simulink model "rc_coder"  (R2019b)
settings: Solver=FixedStepDiscrete  StartTime=0.0  StopTime=Inf  FixedStep=0.025  RelTol=1e-3  EnableMultiTasking=on
PreLoadFcn:
  | mdlname = bdroot;
  | oldFolder = cd(fileparts(which(mdlname)));
  | % cd ..\
  | 
  | load('./bus_type/bus_type.mat');
model workspace (MAT data in the model file):
  ADCDRES : Simulink.Parameter (value not decoded)
  ADCSRES : Simulink.Parameter (value not decoded)
  CLK : Simulink.Parameter (value not decoded)
  EncoderScaler : Simulink.Parameter (value not decoded)
  GearBoxScaler : Simulink.Parameter (value not decoded)
  Kd_T : Simulink.Parameter (value not decoded)
  Kd_theta : Simulink.Parameter (value not decoded)
  Ki_T : Simulink.Parameter (value not decoded)
  Ki_theta : Simulink.Parameter (value not decoded)
  Kp_T : Simulink.Parameter (value not decoded)
  Kp_theta : Simulink.Parameter (value not decoded)
  LowerTempLimitHigh : Simulink.Parameter (value not decoded)
  LowerTempLimitLow : Simulink.Parameter (value not decoded)
  MinMeasurableSpd : Simulink.Parameter (value not decoded)
  ModePWM : Simulink.Parameter (value not decoded)
  ModePosition : Simulink.Parameter (value not decoded)
  ModePrecool : Simulink.Parameter (value not decoded)
  ModeTemp : Simulink.Parameter (value not decoded)
  PWMFreq : Simulink.Parameter (value not decoded)
  QuadratureEncScaler : Simulink.Parameter (value not decoded)
  S1DelaySeconds : Simulink.Parameter (value not decoded)
  S2DelaySeconds : Simulink.Parameter (value not decoded)
  S3DelaySeconds : Simulink.Parameter (value not decoded)
  S4DelaySeconds : Simulink.Parameter (value not decoded)
  SamplingR : Simulink.Parameter (value not decoded)
  StepSize : Simulink.Parameter (value not decoded)
  TErrBand : Simulink.Parameter (value not decoded)
  ThetaErrBand : Simulink.Parameter (value not decoded)
  VADCREF : Simulink.Parameter (value not decoded)
symbols that are objects in the model workspace (value not decoded): ADCDRES, CLK, EncoderScaler, GearBoxScaler, Kd_T, Kd_theta, Ki_T, Ki_theta, Kp_T, Kp_theta, LowerTempLimitHigh, LowerTempLimitLow, MinMeasurableSpd, ModePosition, ModePrecool, ModePWM, ModeTemp, PWMFreq, QuadratureEncScaler, S1DelaySeconds, S2DelaySeconds, S3DelaySeconds, S4DelaySeconds, StepSize, TErrBand, ThetaErrBand
undefined symbols (not defined in the file or in its folder): DiscIntNeverNeededParam, Down, GPTRIP1SEL, GPTRIP2SEL, TZ1, TZ2, Up
libraries: simulink x21, c2802xlib x12, c2837xDlib x10, c280xlib x9, dspstat3 x8, dspfdesign x7, commutil2 x3, c2000lib x2
(part 3 of 4)

== system rc_coder/Sensing/Temperature Measurement/Subsystem ==
  In1 : Inport
  In2 : Inport  Port=2
  In3 : Inport  Port=3
  Divide : Product  Inputs=*/
  Product : Product
  R vs. T : Lookup_n-D  NumberOfTableDimensions=1  BreakpointsForDimension1=|  Table=fliplr([-40:125])  InternalRulePriority=Speed  RndMeth=Simplest  InputSameDT=on
      | flipud([336103
      | 314558
      | 294529
      | 275901
      | 258567
      | 242430
      | 227401
      | 213397
      | 200341
      | 188166
      | 176805
      | 166200
      | 156296
      | 147043
      | 138395
      | 130308
      | 122742
      | 115662
      | 109033
      | 102825
      | 97006.9000000000
      | 91553.3000000000
      | 86439.2000000000
      | 81641.4000000000
      | 77138.6000000000
      | 72911.1000000000
      | 68940.4000000000
      | 65209.7000000000
      | 61702.9000000000
      | 58405.5000000000
      | 55303.9000000000
      | 52385.2000000000
      | 49637.8000000000
      | 47050.6000000000
      | 44613.4000000000
      | 42316.7000000000
      | 40151.6000000000
      | 38110
      | 36184
      | 34366.6000000000
      | 32650.9000000000
      | 31030.8000000000
      | 29500.5000000000
      | 28054.4000000000
      | 26687.5000000000
      | 25395
      | 24172.5000000000
      | 23015.9000000000
      | 21921.2000000000
      | 20884.7000000000
      | 19903.2000000000
      | 18973.3000000000
      | 18092.2000000000
      | 17256.9000000000
      | 16464.9000000000
      | 15713.7000000000
      | 15000.9000000000
      | 14324.5000000000
      | 13682.3000000000
      | 13072.6000000000
      | 12493.3000000000
      | 11943
      | 11419.9000000000
      | 10922.7000000000
      | 10449.8000000000
      | 10000
      | 9572
      | 9164.70000000000
      | 8777
      | 8407.70000000000
      | 8056.10000000000
      | 7721
      | 7401.70000000000
      | 7097.30000000000
      | 6807.10000000000
      | 6530.30000000000
      | 6266.20000000000
      | 6014.30000000000
      | 5773.80000000000
      | 5544.20000000000
      | 5325
      | 5115.60000000000
      | 4915.60000000000
      | 4724.40000000000
      | 4541.70000000000
      | 4367
      | 4200
      | 4040.20000000000
      | 3887.40000000000
      | 3741.10000000000
      | 3601.10000000000
      | 3467
      | 3338.70000000000
      | 3215.80000000000
      | 3098
      | 2985.20000000000
      | 2877
      | 2773.30000000000
      | 2673.90000000000
      | 2578.60000000000
      | 2487.10000000000
      | 2399.40000000000
      | 2315.20000000000
      | 2234.40000000000
      | 2156.80000000000
      | 2082.30000000000
      | 2010.80000000000
      | 1942.10000000000
      | 1876
      | 1812.60000000000
      | 1751.60000000000
      | 1693
      | 1636.60000000000
      | 1582.40000000000
      | 1530.20000000000
      | 1480.10000000000
      | 1431.80000000000
      | 1385.30000000000
      | 1340.60000000000
      | 1297.50000000000
      | 1256.10000000000
      | 1216.10000000000
      | 1177.70000000000
      | 1140.60000000000
      | 1104.90000000000
      | 1070.50000000000
      | 1037.30000000000
      | 1005.30000000000
      | 974.400000000000
      | 944.700000000000
      | 916
      | 888.300000000000
      | 861.500000000000
      | 835.800000000000
      | 810.900000000000
      | 786.800000000000
      | 763.600000000000
      | 741.200000000000
      | 719.600000000000
      | 698.600000000000
      | 678.400000000000
      | 658.900000000000
      | 640
      | 621.800000000000
      | 604.200000000000
      | 587.100000000000
      | 570.600000000000
      | 554.600000000000
      | 539.200000000000
      | 524.300000000000
      | 509.800000000000
      | 495.900000000000
      | 482.300000000000
      | 469.200000000000
      | 456.500000000000
      | 444.200000000000
      | 432.300000000000
      | 420.800000000000
      | 409.700000000000
      | 398.800000000000
      | 388.400000000000
      | 378.200000000000
      | 368.300000000000
      | 358.800000000000
      | 349.500000000000
      | 340.600000000000])
  Subtract : Sum  Inputs=+-
  Out1 : Outport
  wires:
  Product/1 -> Divide/1
  Subtract/1 -> Divide/2
  In3/1 -> Product/2, Subtract/2
  In1/1 -> Subtract/1
  R vs. T/1 -> Out1/1
  In2/1 -> Product/1
  Divide/1 -> R vs. T/1

== system rc_coder/Sensing/Temperature Measurement/Subsystem1 ==
  In1 : Inport
  In2 : Inport  Port=2
  In3 : Inport  Port=3
  Divide : Product  Inputs=*/
  Product : Product
  R vs. T : Lookup_n-D  NumberOfTableDimensions=1  BreakpointsForDimension1=|  Table=fliplr([-40:125])  InternalRulePriority=Speed  RndMeth=Simplest  InputSameDT=on
      | flipud([336103
      | 314558
      | 294529
      | 275901
      | 258567
      | 242430
      | 227401
      | 213397
      | 200341
      | 188166
      | 176805
      | 166200
      | 156296
      | 147043
      | 138395
      | 130308
      | 122742
      | 115662
      | 109033
      | 102825
      | 97006.9000000000
      | 91553.3000000000
      | 86439.2000000000
      | 81641.4000000000
      | 77138.6000000000
      | 72911.1000000000
      | 68940.4000000000
      | 65209.7000000000
      | 61702.9000000000
      | 58405.5000000000
      | 55303.9000000000
      | 52385.2000000000
      | 49637.8000000000
      | 47050.6000000000
      | 44613.4000000000
      | 42316.7000000000
      | 40151.6000000000
      | 38110
      | 36184
      | 34366.6000000000
      | 32650.9000000000
      | 31030.8000000000
      | 29500.5000000000
      | 28054.4000000000
      | 26687.5000000000
      | 25395
      | 24172.5000000000
      | 23015.9000000000
      | 21921.2000000000
      | 20884.7000000000
      | 19903.2000000000
      | 18973.3000000000
      | 18092.2000000000
      | 17256.9000000000
      | 16464.9000000000
      | 15713.7000000000
      | 15000.9000000000
      | 14324.5000000000
      | 13682.3000000000
      | 13072.6000000000
      | 12493.3000000000
      | 11943
      | 11419.9000000000
      | 10922.7000000000
      | 10449.8000000000
      | 10000
      | 9572
      | 9164.70000000000
      | 8777
      | 8407.70000000000
      | 8056.10000000000
      | 7721
      | 7401.70000000000
      | 7097.30000000000
      | 6807.10000000000
      | 6530.30000000000
      | 6266.20000000000
      | 6014.30000000000
      | 5773.80000000000
      | 5544.20000000000
      | 5325
      | 5115.60000000000
      | 4915.60000000000
      | 4724.40000000000
      | 4541.70000000000
      | 4367
      | 4200
      | 4040.20000000000
      | 3887.40000000000
      | 3741.10000000000
      | 3601.10000000000
      | 3467
      | 3338.70000000000
      | 3215.80000000000
      | 3098
      | 2985.20000000000
      | 2877
      | 2773.30000000000
      | 2673.90000000000
      | 2578.60000000000
      | 2487.10000000000
      | 2399.40000000000
      | 2315.20000000000
      | 2234.40000000000
      | 2156.80000000000
      | 2082.30000000000
      | 2010.80000000000
      | 1942.10000000000
      | 1876
      | 1812.60000000000
      | 1751.60000000000
      | 1693
      | 1636.60000000000
      | 1582.40000000000
      | 1530.20000000000
      | 1480.10000000000
      | 1431.80000000000
      | 1385.30000000000
      | 1340.60000000000
      | 1297.50000000000
      | 1256.10000000000
      | 1216.10000000000
      | 1177.70000000000
      | 1140.60000000000
      | 1104.90000000000
      | 1070.50000000000
      | 1037.30000000000
      | 1005.30000000000
      | 974.400000000000
      | 944.700000000000
      | 916
      | 888.300000000000
      | 861.500000000000
      | 835.800000000000
      | 810.900000000000
      | 786.800000000000
      | 763.600000000000
      | 741.200000000000
      | 719.600000000000
      | 698.600000000000
      | 678.400000000000
      | 658.900000000000
      | 640
      | 621.800000000000
      | 604.200000000000
      | 587.100000000000
      | 570.600000000000
      | 554.600000000000
      | 539.200000000000
      | 524.300000000000
      | 509.800000000000
      | 495.900000000000
      | 482.300000000000
      | 469.200000000000
      | 456.500000000000
      | 444.200000000000
      | 432.300000000000
      | 420.800000000000
      | 409.700000000000
      | 398.800000000000
      | 388.400000000000
      | 378.200000000000
      | 368.300000000000
      | 358.800000000000
      | 349.500000000000
      | 340.600000000000])
  Subtract : Sum  Inputs=+-
  Out1 : Outport
  wires:
  Divide/1 -> R vs. T/1
  In2/1 -> Product/1
  R vs. T/1 -> Out1/1
  In1/1 -> Subtract/1
  In3/1 -> Subtract/2, Product/2
  Subtract/1 -> Divide/2
  Product/1 -> Divide/1

== system rc_coder/Sensing/Temperature Measurement/Subsystem2 ==
  In1 : Inport
  In2 : Inport  Port=2
  In3 : Inport  Port=3
  Divide : Product  Inputs=*/
  Product : Product
  R vs. T : Lookup_n-D  NumberOfTableDimensions=1  BreakpointsForDimension1=|  Table=fliplr([-40:125])  InternalRulePriority=Speed  RndMeth=Simplest  InputSameDT=on
      | flipud([336103
      | 314558
      | 294529
      | 275901
      | 258567
      | 242430
      | 227401
      | 213397
      | 200341
      | 188166
      | 176805
      | 166200
      | 156296
      | 147043
      | 138395
      | 130308
      | 122742
      | 115662
      | 109033
      | 102825
      | 97006.9000000000
      | 91553.3000000000
      | 86439.2000000000
      | 81641.4000000000
      | 77138.6000000000
      | 72911.1000000000
      | 68940.4000000000
      | 65209.7000000000
      | 61702.9000000000
      | 58405.5000000000
      | 55303.9000000000
      | 52385.2000000000
      | 49637.8000000000
      | 47050.6000000000
      | 44613.4000000000
      | 42316.7000000000
      | 40151.6000000000
      | 38110
      | 36184
      | 34366.6000000000
      | 32650.9000000000
      | 31030.8000000000
      | 29500.5000000000
      | 28054.4000000000
      | 26687.5000000000
      | 25395
      | 24172.5000000000
      | 23015.9000000000
      | 21921.2000000000
      | 20884.7000000000
      | 19903.2000000000
      | 18973.3000000000
      | 18092.2000000000
      | 17256.9000000000
      | 16464.9000000000
      | 15713.7000000000
      | 15000.9000000000
      | 14324.5000000000
      | 13682.3000000000
      | 13072.6000000000
      | 12493.3000000000
      | 11943
      | 11419.9000000000
      | 10922.7000000000
      | 10449.8000000000
      | 10000
      | 9572
      | 9164.70000000000
      | 8777
      | 8407.70000000000
      | 8056.10000000000
      | 7721
      | 7401.70000000000
      | 7097.30000000000
      | 6807.10000000000
      | 6530.30000000000
      | 6266.20000000000
      | 6014.30000000000
      | 5773.80000000000
      | 5544.20000000000
      | 5325
      | 5115.60000000000
      | 4915.60000000000
      | 4724.40000000000
      | 4541.70000000000
      | 4367
      | 4200
      | 4040.20000000000
      | 3887.40000000000
      | 3741.10000000000
      | 3601.10000000000
      | 3467
      | 3338.70000000000
      | 3215.80000000000
      | 3098
      | 2985.20000000000
      | 2877
      | 2773.30000000000
      | 2673.90000000000
      | 2578.60000000000
      | 2487.10000000000
      | 2399.40000000000
      | 2315.20000000000
      | 2234.40000000000
      | 2156.80000000000
      | 2082.30000000000
      | 2010.80000000000
      | 1942.10000000000
      | 1876
      | 1812.60000000000
      | 1751.60000000000
      | 1693
      | 1636.60000000000
      | 1582.40000000000
      | 1530.20000000000
      | 1480.10000000000
      | 1431.80000000000
      | 1385.30000000000
      | 1340.60000000000
      | 1297.50000000000
      | 1256.10000000000
      | 1216.10000000000
      | 1177.70000000000
      | 1140.60000000000
      | 1104.90000000000
      | 1070.50000000000
      | 1037.30000000000
      | 1005.30000000000
      | 974.400000000000
      | 944.700000000000
      | 916
      | 888.300000000000
      | 861.500000000000
      | 835.800000000000
      | 810.900000000000
      | 786.800000000000
      | 763.600000000000
      | 741.200000000000
      | 719.600000000000
      | 698.600000000000
      | 678.400000000000
      | 658.900000000000
      | 640
      | 621.800000000000
      | 604.200000000000
      | 587.100000000000
      | 570.600000000000
      | 554.600000000000
      | 539.200000000000
      | 524.300000000000
      | 509.800000000000
      | 495.900000000000
      | 482.300000000000
      | 469.200000000000
      | 456.500000000000
      | 444.200000000000
      | 432.300000000000
      | 420.800000000000
      | 409.700000000000
      | 398.800000000000
      | 388.400000000000
      | 378.200000000000
      | 368.300000000000
      | 358.800000000000
      | 349.500000000000
      | 340.600000000000])
  Subtract : Sum  Inputs=+-
  Out1 : Outport
  wires:
  Divide/1 -> R vs. T/1
  In2/1 -> Product/1
  R vs. T/1 -> Out1/1
  In1/1 -> Subtract/1
  In3/1 -> Subtract/2, Product/2
  Subtract/1 -> Divide/2
  Product/1 -> Divide/1

== system rc_coder/Sensing/Temperature Measurement/Subsystem3 ==
  In1 : Inport
  In2 : Inport  Port=2
  In3 : Inport  Port=3
  Divide : Product  Inputs=*/
  Product : Product
  R vs. T : Lookup_n-D  NumberOfTableDimensions=1  BreakpointsForDimension1=|  Table=fliplr([-40:125])  InternalRulePriority=Speed  RndMeth=Simplest  InputSameDT=on
      | flipud([336103
      | 314558
      | 294529
      | 275901
      | 258567
      | 242430
      | 227401
      | 213397
      | 200341
      | 188166
      | 176805
      | 166200
      | 156296
      | 147043
      | 138395
      | 130308
      | 122742
      | 115662
      | 109033
      | 102825
      | 97006.9000000000
      | 91553.3000000000
      | 86439.2000000000
      | 81641.4000000000
      | 77138.6000000000
      | 72911.1000000000
      | 68940.4000000000
      | 65209.7000000000
      | 61702.9000000000
      | 58405.5000000000
      | 55303.9000000000
      | 52385.2000000000
      | 49637.8000000000
      | 47050.6000000000
      | 44613.4000000000
      | 42316.7000000000
      | 40151.6000000000
      | 38110
      | 36184
      | 34366.6000000000
      | 32650.9000000000
      | 31030.8000000000
      | 29500.5000000000
      | 28054.4000000000
      | 26687.5000000000
      | 25395
      | 24172.5000000000
      | 23015.9000000000
      | 21921.2000000000
      | 20884.7000000000
      | 19903.2000000000
      | 18973.3000000000
      | 18092.2000000000
      | 17256.9000000000
      | 16464.9000000000
      | 15713.7000000000
      | 15000.9000000000
      | 14324.5000000000
      | 13682.3000000000
      | 13072.6000000000
      | 12493.3000000000
      | 11943
      | 11419.9000000000
      | 10922.7000000000
      | 10449.8000000000
      | 10000
      | 9572
      | 9164.70000000000
      | 8777
      | 8407.70000000000
      | 8056.10000000000
      | 7721
      | 7401.70000000000
      | 7097.30000000000
      | 6807.10000000000
      | 6530.30000000000
      | 6266.20000000000
      | 6014.30000000000
      | 5773.80000000000
      | 5544.20000000000
      | 5325
      | 5115.60000000000
      | 4915.60000000000
      | 4724.40000000000
      | 4541.70000000000
      | 4367
      | 4200
      | 4040.20000000000
      | 3887.40000000000
      | 3741.10000000000
      | 3601.10000000000
      | 3467
      | 3338.70000000000
      | 3215.80000000000
      | 3098
      | 2985.20000000000
      | 2877
      | 2773.30000000000
      | 2673.90000000000
      | 2578.60000000000
      | 2487.10000000000
      | 2399.40000000000
      | 2315.20000000000
      | 2234.40000000000
      | 2156.80000000000
      | 2082.30000000000
      | 2010.80000000000
      | 1942.10000000000
      | 1876
      | 1812.60000000000
      | 1751.60000000000
      | 1693
      | 1636.60000000000
      | 1582.40000000000
      | 1530.20000000000
      | 1480.10000000000
      | 1431.80000000000
      | 1385.30000000000
      | 1340.60000000000
      | 1297.50000000000
      | 1256.10000000000
      | 1216.10000000000
      | 1177.70000000000
      | 1140.60000000000
      | 1104.90000000000
      | 1070.50000000000
      | 1037.30000000000
      | 1005.30000000000
      | 974.400000000000
      | 944.700000000000
      | 916
      | 888.300000000000
      | 861.500000000000
      | 835.800000000000
      | 810.900000000000
      | 786.800000000000
      | 763.600000000000
      | 741.200000000000
      | 719.600000000000
      | 698.600000000000
      | 678.400000000000
      | 658.900000000000
      | 640
      | 621.800000000000
      | 604.200000000000
      | 587.100000000000
      | 570.600000000000
      | 554.600000000000
      | 539.200000000000
      | 524.300000000000
      | 509.800000000000
      | 495.900000000000
      | 482.300000000000
      | 469.200000000000
      | 456.500000000000
      | 444.200000000000
      | 432.300000000000
      | 420.800000000000
      | 409.700000000000
      | 398.800000000000
      | 388.400000000000
      | 378.200000000000
      | 368.300000000000
      | 358.800000000000
      | 349.500000000000
      | 340.600000000000])
  Subtract : Sum  Inputs=+-
  Out1 : Outport
  wires:
  Divide/1 -> R vs. T/1
  In2/1 -> Product/1
  R vs. T/1 -> Out1/1
  In1/1 -> Subtract/1
  In3/1 -> Subtract/2, Product/2
  Subtract/1 -> Divide/2
  Product/1 -> Divide/1

== system rc_coder/Sensing/Temperature Measurement/exp_formula ==
  note: A power equation with coefficients fitted from offical temperature vs. resistance table.
  In1 : Inport
  In2 : Inport  Port=2
  In3 : Inport  Port=3
  Constant2 : Constant  Value=-0.1445  OutDataTypeStr=double
  Constant3 : Constant  Value=596.8  OutDataTypeStr=double
  Constant4 : Constant  Value=132.8  OutDataTypeStr=double
  Divide : Product  Inputs=*/
  Math Function : Math  Operator=pow  SignedPower=off  SaturateOnIntegerOverflow=on
  Product : Product
  Product1 : Product
  Subtract : Sum  Inputs=+-
  Subtract1 : Sum  Inputs=+-
  Out1 : Outport
  wires:
  In2/1 -> Product/1
  Subtract1/1 -> Out1/1
  In1/1 -> Subtract/1
  Divide/1 -> Math Function/1
  In3/1 -> Subtract/2, Product/2
  Constant4/1 -> Subtract1/2
  Subtract/1 -> Divide/2
  Constant2/1 -> Math Function/2
  Constant3/1 -> Product1/2
  Math Function/1 -> Product1/1
  Product1/1 -> Subtract1/1
  Product/1 -> Divide/1

== system rc_coder/Transmit/DataFlowSwitch/If Action Subsystem1 ==
  Action Port : ActionPort  ActionPortLabel=if((u1 == ModePosition) | (u1 == ModePrecool) | (u1 == ModePWM) | (u1 == ModeTemp))
  Constant : Constant
  Out1 : Outport
  wires:
  Constant/1 -> Out1/1

== system rc_coder/Transmit/DataFlowSwitch/If Action Subsystem2 ==
  In1 : Inport
  Action Port : ActionPort  ActionPortLabel=else
  Compare To Constant1 : simulink/Logic and Bit Operations/Compare To Constant  relop=~=  const=0  OutDataTypeStr=boolean
  Constant3 : Constant  Value=0
  Constant4 : Constant
  Difference : simulink/Discrete/Difference  ICPrevInput=0.0  OutMin=[]  OutMax=[]  OutDataType=fixdt(1, 16)  OutScaling=2^-10  DoSatur=off
  Switch1 : Switch  Criteria=u2 ~= 0
  Out1 : Outport
  wires:
  Switch1/1 -> Out1/1
  Compare To Constant1/1 -> Switch1/2
  In1/1 -> Difference/1
  Constant3/1 -> Switch1/3
  Difference/1 -> Compare To Constant1/1
  Constant4/1 -> Switch1/1

== system rc_coder/Controller/Position Mode/Subsystem1/PID ==
  e : Inport
  Kp : Inport  Port=2
  Ki : Inport  Port=3
  Kd : Inport  Port=4
  Discrete Derivative : simulink/Discrete/Discrete Derivative  gainval=1.0  ICPrevScaledInput=0.0  OutMin=[]  OutMax=[]  OutDataType=fixdt(1, 16)  OutScaling=2^-10  DoSatur=off
  Discrete-Time Integrator : DiscreteIntegrator  SampleTime=-1  LimitOutput=on  UpperSaturationLimit=0.75  LowerSaturationLimit=0  ICPrevOutput=DiscIntNeverNeededParam  ICPrevScaledInput=DiscIntNeverNeededParam
  Product{,1..3} (4 alike) : Product
  Subtract : Sum  Inputs=+++
  error band : Subsystem
  u : Outport
  wires:
  Product3/1 -> u/1
  error band/1(filter) -> Product3/1
  Kp/1 -> Product2/2
  Ki/1 -> Product1/2
  Product1/1 -> Discrete-Time Integrator/1
  Kd/1 -> Product/2
  e/1 -> Product2/1, Product1/1, Product/1, error band/1(e)
  Product/1 -> Discrete Derivative/1
  Product2/1 -> Subtract/1
  Subtract/1 -> Product3/2
  Discrete Derivative/1 -> Subtract/3
  Discrete-Time Integrator/1 -> Subtract/2

== system rc_coder/Controller/Position Mode/Subsystem1/Subsystem ==
  u : Inport
  Constant : Constant  Value=0  OutDataTypeStr=single
  Constant1 : Constant  OutDataTypeStr=single
  Constant2 : Constant  Value=0  OutDataTypeStr=single
  Gain : Gain  Gain=-1
  Switch : Switch  Criteria=u2 > Threshold
  Switch1 : Switch  Criteria=u2 > Threshold
  heating : Outport
  cooling : Outport  Port=2
  wires:
  Constant2/1 -> Switch1/3
  Constant1/1 -> Switch1/1
  Gain/1 -> Switch1/2
  Switch1/1 -> cooling/1
  Constant/1 -> Switch/3
  Switch/1 -> heating/1
  u/1 -> Switch/2, Switch/1, Gain/1

== system rc_coder/Controller/Position Mode/Subsystem2/PID ==
  e : Inport
  Kp : Inport  Port=2
  Ki : Inport  Port=3
  Kd : Inport  Port=4
  Discrete Derivative : simulink/Discrete/Discrete Derivative  gainval=1.0  ICPrevScaledInput=0.0  OutMin=[]  OutMax=[]  OutDataType=fixdt(1, 16)  OutScaling=2^-10  DoSatur=off
  Discrete-Time Integrator : DiscreteIntegrator  SampleTime=-1  LimitOutput=on  UpperSaturationLimit=0.75  LowerSaturationLimit=0  ICPrevOutput=DiscIntNeverNeededParam  ICPrevScaledInput=DiscIntNeverNeededParam
  Product{,1..3} (4 alike) : Product
  Subtract : Sum  Inputs=+++
  error band : Subsystem
  u : Outport
  wires:
  Discrete-Time Integrator/1 -> Subtract/2
  Discrete Derivative/1 -> Subtract/3
  Subtract/1 -> Product3/2
  Product2/1 -> Subtract/1
  Product/1 -> Discrete Derivative/1
  e/1 -> error band/1(e), Product/1, Product1/1, Product2/1
  Kd/1 -> Product/2
  Product1/1 -> Discrete-Time Integrator/1
  Ki/1 -> Product1/2
  Kp/1 -> Product2/2
  error band/1(filter) -> Product3/1
  Product3/1 -> u/1

== system rc_coder/Controller/Position Mode/Subsystem2/Subsystem ==
  u : Inport
  Constant : Constant  Value=0  OutDataTypeStr=single
  Constant1 : Constant  OutDataTypeStr=single
  Constant2 : Constant  Value=0  OutDataTypeStr=single
  Gain : Gain  Gain=-1
  Switch : Switch  Criteria=u2 > Threshold
  Switch1 : Switch  Criteria=u2 > Threshold
  heating : Outport
  cooling : Outport  Port=2
  wires:
  u/1 -> Gain/1, Switch/1, Switch/2
  Switch/1 -> heating/1
  Constant/1 -> Switch/3
  Switch1/1 -> cooling/1
  Gain/1 -> Switch1/2
  Constant1/1 -> Switch1/1
  Constant2/1 -> Switch1/3

== system rc_coder/Controller/Position Mode/Subsystem3/PID ==
  e : Inport
  Kp : Inport  Port=2
  Ki : Inport  Port=3
  Kd : Inport  Port=4
  Discrete Derivative : simulink/Discrete/Discrete Derivative  gainval=1.0  ICPrevScaledInput=0.0  OutMin=[]  OutMax=[]  OutDataType=fixdt(1, 16)  OutScaling=2^-10  DoSatur=off
  Discrete-Time Integrator : DiscreteIntegrator  SampleTime=-1  LimitOutput=on  UpperSaturationLimit=0.75  LowerSaturationLimit=0  ICPrevOutput=DiscIntNeverNeededParam  ICPrevScaledInput=DiscIntNeverNeededParam
  Product{,1..3} (4 alike) : Product
  Subtract : Sum  Inputs=+++
  error band : Subsystem
  u : Outport
  wires:
  Discrete-Time Integrator/1 -> Subtract/2
  Discrete Derivative/1 -> Subtract/3
  Subtract/1 -> Product3/2
  Product2/1 -> Subtract/1
  Product/1 -> Discrete Derivative/1
  e/1 -> error band/1(e), Product/1, Product1/1, Product2/1
  Kd/1 -> Product/2
  Product1/1 -> Discrete-Time Integrator/1
  Ki/1 -> Product1/2
  Kp/1 -> Product2/2
  error band/1(filter) -> Product3/1
  Product3/1 -> u/1

== system rc_coder/Controller/Position Mode/Subsystem3/Subsystem ==
  u : Inport
  Constant : Constant  Value=0  OutDataTypeStr=single
  Constant1 : Constant  OutDataTypeStr=single
  Constant2 : Constant  Value=0  OutDataTypeStr=single
  Gain : Gain  Gain=-1
  Switch : Switch  Criteria=u2 > Threshold
  Switch1 : Switch  Criteria=u2 > Threshold
  heating : Outport
  cooling : Outport  Port=2
  wires:
  u/1 -> Gain/1, Switch/1, Switch/2
  Switch/1 -> heating/1
  Constant/1 -> Switch/3
  Switch1/1 -> cooling/1
  Gain/1 -> Switch1/2
  Constant1/1 -> Switch1/1
  Constant2/1 -> Switch1/3

== system rc_coder/Controller/Position Mode/Subsystem4/PID ==
  e : Inport
  Kp : Inport  Port=2
  Ki : Inport  Port=3
  Kd : Inport  Port=4
  Discrete Derivative : simulink/Discrete/Discrete Derivative  gainval=1.0  ICPrevScaledInput=0.0  OutMin=[]  OutMax=[]  OutDataType=fixdt(1, 16)  OutScaling=2^-10  DoSatur=off
  Discrete-Time Integrator : DiscreteIntegrator  SampleTime=-1  LimitOutput=on  UpperSaturationLimit=0.75  LowerSaturationLimit=0  ICPrevOutput=DiscIntNeverNeededParam  ICPrevScaledInput=DiscIntNeverNeededParam
  Product{,1..3} (4 alike) : Product
  Subtract : Sum  Inputs=+++
  error band : Subsystem
  u : Outport
  wires:
  Product3/1 -> u/1
  error band/1(filter) -> Product3/1
  Kp/1 -> Product2/2
  Ki/1 -> Product1/2
  Product1/1 -> Discrete-Time Integrator/1
  Kd/1 -> Product/2
  e/1 -> Product2/1, Product1/1, Product/1, error band/1(e)
  Product/1 -> Discrete Derivative/1
  Product2/1 -> Subtract/1
  Subtract/1 -> Product3/2
  Discrete Derivative/1 -> Subtract/3
  Discrete-Time Integrator/1 -> Subtract/2

== system rc_coder/Controller/Position Mode/Subsystem4/Subsystem ==
  u : Inport
  Constant : Constant  Value=0  OutDataTypeStr=single
  Constant1 : Constant  OutDataTypeStr=single
  Constant2 : Constant  Value=0  OutDataTypeStr=single
  Gain : Gain  Gain=-1
  Switch : Switch  Criteria=u2 > Threshold
  Switch1 : Switch  Criteria=u2 > Threshold
  heating : Outport
  cooling : Outport  Port=2
  wires:
  Constant2/1 -> Switch1/3
  Constant1/1 -> Switch1/1
  Gain/1 -> Switch1/2
  Switch1/1 -> cooling/1
  Constant/1 -> Switch/3
  Switch/1 -> heating/1
  u/1 -> Switch/2, Switch/1, Gain/1

== system rc_coder/Controller/Position Mode/Subsystem5/Subsystem ==
  In1 : Inport
  Add : Sum
  Constant : Constant  Value=44
  Constant1 : Constant  Value=42.8554
  d2T : Gain  Gain=1 / 2.3178
  theta2displacement : Gain  Gain=1 / 360 * 2 * pi * 5.2
  Out1 : Outport
  wires:
  In1/1 -> theta2displacement/1
  Constant/1 -> Add/2
  d2T/1 -> Add/1
  theta2displacement/1 -> d2T/1
  Add/1 -> Out1/1

== system rc_coder/Controller/Position Mode/Subsystem5/Subsystem1 ==
  In1 : Inport
  Add : Sum
  Constant : Constant  Value=42.8554
  d2T : Gain  Gain=1 / 2.3178
  theta2displacement : Gain  Gain=1 / 360 * 2 * pi * 5.2
  Out1 : Outport
  wires:
  Add/1 -> Out1/1
  theta2displacement/1 -> d2T/1
  d2T/1 -> Add/1
  Constant/1 -> Add/2
  In1/1 -> theta2displacement/1

== system rc_coder/Controller/Position Mode/Subsystem5/Subsystem2 ==
  delay s : Inport
  Constant : Constant  Value=LowerTempLimitHigh
  Constant1 : Constant  Value=LowerTempLimitLow
  Delay : Delay  DelayLengthSource=Input port  DelayLengthUpperLimit=500  InitialConditionSource=Input port
      settings: InputPortMap=u0,p1,p4
  Gain : Gain  Gain=1 / StepSize
  lower limit : Outport
  wires:
  delay s/1 -> Gain/1
  Gain/1 -> Delay/2
  Constant/1 -> Delay/1
  Constant1/1 -> Delay/3
  Delay/1 -> lower limit/1

== system rc_coder/Controller/Position Mode/Subsystem5/Subsystem3 ==
  delay s : Inport
  Constant : Constant  Value=LowerTempLimitHigh
  Constant1 : Constant  Value=LowerTempLimitLow
  Delay : Delay  DelayLengthSource=Input port  DelayLengthUpperLimit=500  InitialConditionSource=Input port
      settings: InputPortMap=u0,p1,p4
  Gain : Gain  Gain=1 / StepSize
  lower limit : Outport
  wires:
  Delay/1 -> lower limit/1
  Constant1/1 -> Delay/3
  Constant/1 -> Delay/1
  Gain/1 -> Delay/2
  delay s/1 -> Gain/1

== system rc_coder/Controller/Position Mode/Subsystem5/feedforward1 ==
  d : Inport
  Add : Sum  Inputs=++-
  Add1 : Sum
  Constant : Constant  Value=0.01146
  Constant1 : Constant  Value=40
  Constant3 : Constant  Value=30
  Gain : Gain  Gain=0.001
  Gain1 : Gain  Gain=707.6
  Gain2 : Gain  Gain=36.25
  Math Function : Math  Operator=pow  SignedPower=off  SaturateOnIntegerOverflow=on
  T : Outport
  wires:
  Gain/1 -> Math Function/1, Gain1/1
  Constant1/1 -> Add1/2
  d/1 -> Add1/1
  Constant3/1 -> Add/3
  Add1/1 -> Gain/1
  Add/1 -> T/1
  Gain1/1 -> Add/1
  Gain2/1 -> Add/2
  Math Function/1 -> Gain2/1
  Constant/1 -> Math Function/2

== system rc_coder/Controller/Position Mode/Subsystem6/Subsystem ==
  In1 : Inport
  Add : Sum
  Constant : Constant  Value=44
  Constant1 : Constant  Value=42.8554
  d2T : Gain  Gain=1 / 2.3178
  theta2displacement : Gain  Gain=1 / 360 * 2 * pi * 5.2
  Out1 : Outport
  wires:
  Add/1 -> Out1/1
  theta2displacement/1 -> d2T/1
  d2T/1 -> Add/1
  Constant/1 -> Add/2
  In1/1 -> theta2displacement/1

== system rc_coder/Controller/Position Mode/Subsystem6/Subsystem1 ==
  In1 : Inport
  Add : Sum
  Constant : Constant  Value=42.8554
  d2T : Gain  Gain=1 / 2.3178
  theta2displacement : Gain  Gain=1 / 360 * 2 * pi * 5.2
  Out1 : Outport
  wires:
  In1/1 -> theta2displacement/1
  Constant/1 -> Add/2
  d2T/1 -> Add/1
  theta2displacement/1 -> d2T/1
  Add/1 -> Out1/1

== system rc_coder/Controller/Position Mode/Subsystem6/Subsystem2 ==
  delay s : Inport
  Constant : Constant  Value=LowerTempLimitHigh
  Constant1 : Constant  Value=LowerTempLimitLow
  Delay : Delay  DelayLengthSource=Input port  DelayLengthUpperLimit=500  InitialConditionSource=Input port
      settings: InputPortMap=u0,p1,p4
  Gain : Gain  Gain=1 / StepSize
  lower limit : Outport
  wires:
  delay s/1 -> Gain/1
  Gain/1 -> Delay/2
  Constant/1 -> Delay/1
  Constant1/1 -> Delay/3
  Delay/1 -> lower limit/1

== system rc_coder/Controller/Position Mode/Subsystem6/Subsystem3 ==
  delay s : Inport
  Constant : Constant  Value=LowerTempLimitHigh
  Constant1 : Constant  Value=LowerTempLimitLow
  Delay : Delay  DelayLengthSource=Input port  DelayLengthUpperLimit=500  InitialConditionSource=Input port
      settings: InputPortMap=u0,p1,p4
  Gain : Gain  Gain=1 / StepSize
  lower limit : Outport
  wires:
  delay s/1 -> Gain/1
  Gain/1 -> Delay/2
  Constant/1 -> Delay/1
  Constant1/1 -> Delay/3
  Delay/1 -> lower limit/1

== system rc_coder/Controller/Position Mode/Subsystem6/feedforward1 ==
  d : Inport
  Add : Sum  Inputs=++-
  Add1 : Sum
  Constant : Constant  Value=0.01146
  Constant1 : Constant  Value=40
  Constant3 : Constant  Value=30
  Gain : Gain  Gain=0.001
  Gain1 : Gain  Gain=707.6
  Gain2 : Gain  Gain=36.25
  Math Function : Math  Operator=pow  SignedPower=off  SaturateOnIntegerOverflow=on
  T : Outport
  wires:
  Constant/1 -> Math Function/2
  Math Function/1 -> Gain2/1
  Gain2/1 -> Add/2
  Gain1/1 -> Add/1
  Add/1 -> T/1
  Add1/1 -> Gain/1
  Constant3/1 -> Add/3
  d/1 -> Add1/1
  Constant1/1 -> Add1/2
  Gain/1 -> Gain1/1, Math Function/1

== system rc_coder/Controller/Temperature Mode/Subsystem1/PID ==
  e : Inport
  Kp : Inport  Port=2
  Ki : Inport  Port=3
  Kd : Inport  Port=4
  Discrete Derivative : simulink/Discrete/Discrete Derivative  gainval=1.0  ICPrevScaledInput=0.0  OutMin=[]  OutMax=[]  OutDataType=fixdt(1, 16)  OutScaling=2^-10  DoSatur=off
  Discrete-Time Integrator : DiscreteIntegrator  SampleTime=-1  LimitOutput=on  UpperSaturationLimit=0.75  LowerSaturationLimit=0  ICPrevOutput=DiscIntNeverNeededParam  ICPrevScaledInput=DiscIntNeverNeededParam
  Product{,1..3} (4 alike) : Product
  Subtract : Sum  Inputs=+++
  error band : Subsystem
  u : Outport
  wires:
  Discrete-Time Integrator/1 -> Subtract/2
  Discrete Derivative/1 -> Subtract/3
  Subtract/1 -> Product3/2
  Product2/1 -> Subtract/1
  Product/1 -> Discrete Derivative/1
  e/1 -> error band/1(e), Product/1, Product1/1, Product2/1
  Kd/1 -> Product/2
  Product1/1 -> Discrete-Time Integrator/1
  Ki/1 -> Product1/2
  Kp/1 -> Product2/2
  error band/1(filter) -> Product3/1
  Product3/1 -> u/1

== system rc_coder/Controller/Temperature Mode/Subsystem1/Subsystem ==
  u : Inport
  Constant : Constant  Value=0  OutDataTypeStr=single
  Constant1 : Constant  OutDataTypeStr=single
  Constant2 : Constant  Value=0  OutDataTypeStr=single
  Gain : Gain  Gain=-1
  Switch : Switch  Criteria=u2 > Threshold
  Switch1 : Switch  Criteria=u2 > Threshold
  heating : Outport
  cooling : Outport  Port=2
  wires:
  u/1 -> Gain/1, Switch/1, Switch/2
  Switch/1 -> heating/1
  Constant/1 -> Switch/3
  Switch1/1 -> cooling/1
  Gain/1 -> Switch1/2
  Constant1/1 -> Switch1/1
  Constant2/1 -> Switch1/3

== system rc_coder/Controller/Temperature Mode/Subsystem2/PID ==
  e : Inport
  Kp : Inport  Port=2
  Ki : Inport  Port=3
  Kd : Inport  Port=4
  Discrete Derivative : simulink/Discrete/Discrete Derivative  gainval=1.0  ICPrevScaledInput=0.0  OutMin=[]  OutMax=[]  OutDataType=fixdt(1, 16)  OutScaling=2^-10  DoSatur=off
  Discrete-Time Integrator : DiscreteIntegrator  SampleTime=-1  LimitOutput=on  UpperSaturationLimit=0.75  LowerSaturationLimit=0  ICPrevOutput=DiscIntNeverNeededParam  ICPrevScaledInput=DiscIntNeverNeededParam
  Product{,1..3} (4 alike) : Product
  Subtract : Sum  Inputs=+++
  error band : Subsystem
  u : Outport
  wires:
  Product3/1 -> u/1
  error band/1(filter) -> Product3/1
  Kp/1 -> Product2/2
  Ki/1 -> Product1/2
  Product1/1 -> Discrete-Time Integrator/1
  Kd/1 -> Product/2
  e/1 -> Product2/1, Product1/1, Product/1, error band/1(e)
  Product/1 -> Discrete Derivative/1
  Product2/1 -> Subtract/1
  Subtract/1 -> Product3/2
  Discrete Derivative/1 -> Subtract/3
  Discrete-Time Integrator/1 -> Subtract/2

== system rc_coder/Controller/Temperature Mode/Subsystem2/Subsystem ==
  u : Inport
  Constant : Constant  Value=0  OutDataTypeStr=single
  Constant1 : Constant  OutDataTypeStr=single
  Constant2 : Constant  Value=0  OutDataTypeStr=single
  Gain : Gain  Gain=-1
  Switch : Switch  Criteria=u2 > Threshold
  Switch1 : Switch  Criteria=u2 > Threshold
  heating : Outport
  cooling : Outport  Port=2
  wires:
  Constant2/1 -> Switch1/3
  Constant1/1 -> Switch1/1
  Gain/1 -> Switch1/2
  Switch1/1 -> cooling/1
  Constant/1 -> Switch/3
  Switch/1 -> heating/1
  u/1 -> Switch/2, Switch/1, Gain/1

== system rc_coder/Controller/Temperature Mode/Subsystem3/PID ==
  e : Inport
  Kp : Inport  Port=2
  Ki : Inport  Port=3
  Kd : Inport  Port=4
  Discrete Derivative : simulink/Discrete/Discrete Derivative  gainval=1.0  ICPrevScaledInput=0.0  OutMin=[]  OutMax=[]  OutDataType=fixdt(1, 16)  OutScaling=2^-10  DoSatur=off
  Discrete-Time Integrator : DiscreteIntegrator  SampleTime=-1  LimitOutput=on  UpperSaturationLimit=0.75  LowerSaturationLimit=0  ICPrevOutput=DiscIntNeverNeededParam  ICPrevScaledInput=DiscIntNeverNeededParam
  Product{,1..3} (4 alike) : Product
  Subtract : Sum  Inputs=+++
  error band : Subsystem
  u : Outport
  wires:
  Product3/1 -> u/1
  error band/1(filter) -> Product3/1
  Kp/1 -> Product2/2
  Ki/1 -> Product1/2
  Product1/1 -> Discrete-Time Integrator/1
  Kd/1 -> Product/2
  e/1 -> Product2/1, Product1/1, Product/1, error band/1(e)
  Product/1 -> Discrete Derivative/1
  Product2/1 -> Subtract/1
  Subtract/1 -> Product3/2
  Discrete Derivative/1 -> Subtract/3
  Discrete-Time Integrator/1 -> Subtract/2

== system rc_coder/Controller/Temperature Mode/Subsystem3/Subsystem ==
  u : Inport
  Constant : Constant  Value=0  OutDataTypeStr=single
  Constant1 : Constant  OutDataTypeStr=single
  Constant2 : Constant  Value=0  OutDataTypeStr=single
  Gain : Gain  Gain=-1
  Switch : Switch  Criteria=u2 > Threshold
  Switch1 : Switch  Criteria=u2 > Threshold
  heating : Outport
  cooling : Outport  Port=2
  wires:
  Constant2/1 -> Switch1/3
  Constant1/1 -> Switch1/1
  Gain/1 -> Switch1/2
  Switch1/1 -> cooling/1
  Constant/1 -> Switch/3
  Switch/1 -> heating/1
  u/1 -> Switch/2, Switch/1, Gain/1

== system rc_coder/Controller/Temperature Mode/Subsystem4/PID ==
  e : Inport
  Kp : Inport  Port=2
  Ki : Inport  Port=3
  Kd : Inport  Port=4
  Discrete Derivative : simulink/Discrete/Discrete Derivative  gainval=1.0  ICPrevScaledInput=0.0  OutMin=[]  OutMax=[]  OutDataType=fixdt(1, 16)  OutScaling=2^-10  DoSatur=off
  Discrete-Time Integrator : DiscreteIntegrator  SampleTime=-1  LimitOutput=on  UpperSaturationLimit=0.75  LowerSaturationLimit=0  ICPrevOutput=DiscIntNeverNeededParam  ICPrevScaledInput=DiscIntNeverNeededParam
  Product{,1..3} (4 alike) : Product
  Subtract : Sum  Inputs=+++
  error band : Subsystem
  u : Outport
  wires:
  Discrete-Time Integrator/1 -> Subtract/2
  Discrete Derivative/1 -> Subtract/3
  Subtract/1 -> Product3/2
  Product2/1 -> Subtract/1
  Product/1 -> Discrete Derivative/1
  e/1 -> error band/1(e), Product/1, Product1/1, Product2/1
  Kd/1 -> Product/2
  Product1/1 -> Discrete-Time Integrator/1
  Ki/1 -> Product1/2
  Kp/1 -> Product2/2
  error band/1(filter) -> Product3/1
  Product3/1 -> u/1

== system rc_coder/Controller/Temperature Mode/Subsystem4/Subsystem ==
  u : Inport
  Constant : Constant  Value=0  OutDataTypeStr=single
  Constant1 : Constant  OutDataTypeStr=single
  Constant2 : Constant  Value=0  OutDataTypeStr=single
  Gain : Gain  Gain=-1
  Switch : Switch  Criteria=u2 > Threshold
  Switch1 : Switch  Criteria=u2 > Threshold
  heating : Outport
  cooling : Outport  Port=2
  wires:
  u/1 -> Gain/1, Switch/1, Switch/2
  Switch/1 -> heating/1
  Constant/1 -> Switch/3
  Switch1/1 -> cooling/1
  Gain/1 -> Switch1/2
  Constant1/1 -> Switch1/1
  Constant2/1 -> Switch1/3

== system rc_coder/Controller/Temperature Mode/Subsystem5/PID_1 ==
  e : Inport
  Kp : Inport  Port=2
  Ki : Inport  Port=3
  Kd : Inport  Port=4
  Discrete Derivative : simulink/Discrete/Discrete Derivative  gainval=1.0  ICPrevScaledInput=0.0  OutMin=[]  OutMax=[]  OutDataType=fixdt(1, 16)  OutScaling=2^-10  DoSatur=off
  Discrete-Time Integrator : DiscreteIntegrator  SampleTime=-1  LimitOutput=on  UpperSaturationLimit=0.75  LowerSaturationLimit=0  ICPrevOutput=DiscIntNeverNeededParam  ICPrevScaledInput=DiscIntNeverNeededParam
  Product{,1..3} (4 alike) : Product
  Subtract : Sum  Inputs=+++
  error band : Subsystem
  u : Outport
  wires:
  Product3/1 -> u/1
  error band/1(filter) -> Product3/1
  Kp/1 -> Product2/2
  Ki/1 -> Product1/2
  Product1/1 -> Discrete-Time Integrator/1
  Kd/1 -> Product/2
  e/1 -> Product2/1, Product1/1, Product/1, error band/1(e)
  Product/1 -> Discrete Derivative/1
  Product2/1 -> Subtract/1
  Subtract/1 -> Product3/2
  Discrete Derivative/1 -> Subtract/3
  Discrete-Time Integrator/1 -> Subtract/2

== system rc_coder/Controller/Temperature Mode/Subsystem5/Subsystem ==
  u : Inport
  Constant : Constant  Value=0  OutDataTypeStr=single
  Constant1 : Constant  OutDataTypeStr=single
  Constant2 : Constant  Value=0  OutDataTypeStr=single
  Gain : Gain  Gain=-1
  Switch : Switch  Criteria=u2 > Threshold
  Switch1 : Switch  Criteria=u2 > Threshold
  heating : Outport
  cooling : Outport  Port=2
  wires:
  Constant2/1 -> Switch1/3
  Constant1/1 -> Switch1/1
  Gain/1 -> Switch1/2
  Switch1/1 -> cooling/1
  Constant/1 -> Switch/3
  Switch/1 -> heating/1
  u/1 -> Switch/2, Switch/1, Gain/1

== system rc_coder/Sensing/Incremental Encoder/CalcSpd/OF_Initial_check ==
  spd_in : Inport
  cnt_prd : Inport  Port=2
  OF_flag : Inport  Port=3
  Constant3 : Constant  Value=0
  Constant4 : Constant  Value=0
  Switch2 : Switch  Criteria=u2 ~= 0
  Switch3 : Switch  Criteria=u2 ~= 0
  spd_out : Outport
  wires:
  spd_in/1 -> Switch2/3
  Constant3/1 -> Switch2/1
  Constant4/1 -> Switch3/3
  Switch3/1 -> spd_out/1
  Switch2/1 -> Switch3/1
  cnt_prd/1 -> Switch3/2
  OF_flag/1 -> Switch2/2

== system rc_coder/Sensing/Incremental Encoder/CalcSpd/cnt2rpm ==
  cnt_prd : Inport
  Constant : Constant  Value=(2 * pi) / (EncoderScaler / QuadratureEncScaler * GearBoxScaler)
  Divide : Product  Inputs=/*
  Gain : Gain  Gain=1/CLK  OutDataTypeStr=single
  radps : Outport
  wires:
  Constant/1 -> Divide/2
  cnt_prd/1 -> Gain/1
  Gain/1 -> Divide/1
  Divide/1 -> radps/1

== system rc_coder/Sensing/Incremental Encoder/CalcSpd/dir_check ==
  dir_flag : Inport
  Constant1 : Constant
  Constant2 : Constant  Value=-1
  Switch1 : Switch  Criteria=u2 ~= 0
  dir : Outport
  wires:
  Constant1/1 -> Switch1/1
  Constant2/1 -> Switch1/3
  dir_flag/1 -> Switch1/2
  Switch1/1 -> dir/1

== system rc_coder/Sensing/Incremental Encoder/CalcSpd/zero_spd_check ==
  poscnt : Inport
  last_measurement : Inport  Port=2
  Relational Operator : RelationalOperator  Operator=>  OutDataTypeStr=boolean  RndMeth=Simplest
  Subsystem : Subsystem
  Subsystem1 : Subsystem
  flag : Outport
  wires:
  Subsystem/1(no_measurement_cnt) -> Relational Operator/1
  Subsystem1/1(cnts_to_wait) -> Relational Operator/2
  last_measurement/1 -> Subsystem1/1(spd_last_measurement)
  Relational Operator/1 -> flag/1
  poscnt/1 -> Subsystem/1(poscnt)

== system rc_coder/Sensing/Incremental Encoder/CalcSpd1/OF_Initial_check ==
  spd_in : Inport
  cnt_prd : Inport  Port=2
  OF_flag : Inport  Port=3
  Constant3 : Constant  Value=0
  Constant4 : Constant  Value=0
  Switch2 : Switch  Criteria=u2 ~= 0
  Switch3 : Switch  Criteria=u2 ~= 0
  spd_out : Outport
  wires:
  OF_flag/1 -> Switch2/2
  cnt_prd/1 -> Switch3/2
  Switch2/1 -> Switch3/1
  Switch3/1 -> spd_out/1
  Constant4/1 -> Switch3/3
  Constant3/1 -> Switch2/1
  spd_in/1 -> Switch2/3

== system rc_coder/Sensing/Incremental Encoder/CalcSpd1/cnt2rpm ==
  cnt_prd : Inport
  Constant : Constant  Value=(2 * pi) / (EncoderScaler / QuadratureEncScaler * GearBoxScaler)
  Divide : Product  Inputs=/*
  Gain : Gain  Gain=1/CLK  OutDataTypeStr=single
  radps : Outport
  wires:
  Divide/1 -> radps/1
  Gain/1 -> Divide/1
  cnt_prd/1 -> Gain/1
  Constant/1 -> Divide/2

== system rc_coder/Sensing/Incremental Encoder/CalcSpd1/dir_check ==
  dir_flag : Inport
  Constant1 : Constant
  Constant2 : Constant  Value=-1
  Switch1 : Switch  Criteria=u2 ~= 0
  dir : Outport
  wires:
  Switch1/1 -> dir/1
  dir_flag/1 -> Switch1/2
  Constant2/1 -> Switch1/3
  Constant1/1 -> Switch1/1

== system rc_coder/Sensing/Incremental Encoder/CalcSpd1/zero_spd_check ==
  poscnt : Inport
  last_measurement : Inport  Port=2
  Relational Operator : RelationalOperator  Operator=>  OutDataTypeStr=boolean  RndMeth=Simplest
  Subsystem : Subsystem
  Subsystem1 : Subsystem
  flag : Outport
  wires:
  poscnt/1 -> Subsystem/1(poscnt)
  Relational Operator/1 -> flag/1
  last_measurement/1 -> Subsystem1/1(spd_last_measurement)
  Subsystem1/1(cnts_to_wait) -> Relational Operator/2
  Subsystem/1(no_measurement_cnt) -> Relational Operator/1

== system rc_coder/Controller/Position Mode/Subsystem1/PID/error band ==
  e : Inport
  Abs : Abs
  Constant : Constant
  Constant1 : Constant  Value=0
  Switch : Switch  Criteria=u2 > Threshold  Threshold=TErrBand
  filter : Outport
  wires:
  Switch/1 -> filter/1
  Abs/1 -> Switch/2
  Constant/1 -> Switch/1
  e/1 -> Abs/1
  Constant1/1 -> Switch/3

== system rc_coder/Controller/Position Mode/Subsystem2/PID/error band ==
  e : Inport
  Abs : Abs
  Constant : Constant
  Constant1 : Constant  Value=0
  Switch : Switch  Criteria=u2 > Threshold  Threshold=TErrBand
  filter : Outport
  wires:
  Constant1/1 -> Switch/3
  e/1 -> Abs/1
  Constant/1 -> Switch/1
  Abs/1 -> Switch/2
  Switch/1 -> filter/1

== system rc_coder/Controller/Position Mode/Subsystem3/PID/error band ==
  e : Inport
  Abs : Abs
  Constant : Constant
  Constant1 : Constant  Value=0
  Switch : Switch  Criteria=u2 > Threshold  Threshold=TErrBand
  filter : Outport
  wires:
  Constant1/1 -> Switch/3
  e/1 -> Abs/1
  Constant/1 -> Switch/1
  Abs/1 -> Switch/2
  Switch/1 -> filter/1

== system rc_coder/Controller/Position Mode/Subsystem4/PID/error band ==
  e : Inport
  Abs : Abs
  Constant : Constant
  Constant1 : Constant  Value=0
  Switch : Switch  Criteria=u2 > Threshold  Threshold=TErrBand
  filter : Outport
  wires:
  Switch/1 -> filter/1
  Abs/1 -> Switch/2
  Constant/1 -> Switch/1
  e/1 -> Abs/1
  Constant1/1 -> Switch/3

== system rc_coder/Controller/Temperature Mode/Subsystem1/PID/error band ==
  e : Inport
  Abs : Abs
  Constant : Constant
  Constant1 : Constant  Value=0
  Switch : Switch  Criteria=u2 > Threshold  Threshold=TErrBand
  filter : Outport
  wires:
  Constant1/1 -> Switch/3
  e/1 -> Abs/1
  Constant/1 -> Switch/1
  Abs/1 -> Switch/2
  Switch/1 -> filter/1

== system rc_coder/Controller/Temperature Mode/Subsystem2/PID/error band ==
  e : Inport
  Abs : Abs
  Constant : Constant
  Constant1 : Constant  Value=0
  Switch : Switch  Criteria=u2 > Threshold  Threshold=TErrBand
  filter : Outport
  wires:
  Switch/1 -> filter/1
  Abs/1 -> Switch/2
  Constant/1 -> Switch/1
  e/1 -> Abs/1
  Constant1/1 -> Switch/3

== system rc_coder/Controller/Temperature Mode/Subsystem3/PID/error band ==
  e : Inport
  Abs : Abs
  Constant : Constant
  Constant1 : Constant  Value=0
  Switch : Switch  Criteria=u2 > Threshold  Threshold=TErrBand
  filter : Outport
  wires:
  Switch/1 -> filter/1
  Abs/1 -> Switch/2
  Constant/1 -> Switch/1
  e/1 -> Abs/1
  Constant1/1 -> Switch/3

== system rc_coder/Controller/Temperature Mode/Subsystem4/PID/error band ==
  e : Inport
  Abs : Abs
  Constant : Constant
  Constant1 : Constant  Value=0
  Switch : Switch  Criteria=u2 > Threshold  Threshold=TErrBand
  filter : Outport
  wires:
  Constant1/1 -> Switch/3
  e/1 -> Abs/1
  Constant/1 -> Switch/1
  Abs/1 -> Switch/2
  Switch/1 -> filter/1

== system rc_coder/Controller/Temperature Mode/Subsystem5/PID_1/error band ==
  e : Inport
  Abs : Abs
  Constant : Constant
  Constant1 : Constant  Value=0
  Switch : Switch  Criteria=u2 > Threshold  Threshold=0.1
  filter : Outport
  wires:
  Switch/1 -> filter/1
  Abs/1 -> Switch/2
  Constant/1 -> Switch/1
  e/1 -> Abs/1
  Constant1/1 -> Switch/3

== system rc_coder/Sensing/Incremental Encoder/CalcSpd/zero_spd_check/Subsystem ==
  poscnt : Inport
  Detect Change : simulink/Logic and Bit Operations/Detect Change  vinit=0  OutDataTypeStr=boolean
  If : If  IfExpression=u1 == 1
  If Action Subsystem : Subsystem  TreatAsAtomicUnit=on
  If Action Subsystem1 : Subsystem  TreatAsAtomicUnit=on
  Merge : Merge
  Saturation : Saturate  UpperLimit=60 / (MinMeasurableSpd * EncoderScaler) / StepSize +100  LowerLimit=0
  Unit Delay1 : UnitDelay  SampleTime=-1  HasFrameUpgradeWarning=on
  no_measurement_cnt : Outport
  wires:
  Merge/1 -> Unit Delay1/1, Saturation/1
  Detect Change/1 -> If/1
  Unit Delay1/1 -> If Action Subsystem1/1(In1)
  If Action Subsystem/1(Out1) -> Merge/1
  If Action Subsystem1/1(Out1) -> Merge/2
  If/2 -> If Action Subsystem1/Action
  If/1 -> If Action Subsystem/Action
  poscnt/1 -> Detect Change/1
  Saturation/1 -> no_measurement_cnt/1

== system rc_coder/Sensing/Incremental Encoder/CalcSpd/zero_spd_check/Subsystem1 ==
  spd_last_measurement : Inport
  Constant1 : Constant  Value=60 / (MinMeasurableSpd * EncoderScaler)
  Constant5 : Constant  Value=2 * pi / EncoderScaler
  Divide2 : Product  Inputs=*/
  Gain : Gain  Gain=1 / StepSize
  MinMax : MinMax  Inputs=2
  cnts_to_wait : Outport
  wires:
  Constant5/1 -> Divide2/1
  spd_last_measurement/1 -> Divide2/2
  Divide2/1 -> MinMax/1
  Gain/1 -> cnts_to_wait/1
  MinMax/1 -> Gain/1
  Constant1/1 -> MinMax/2
